simulink model "lab2"  (R2018b)
settings: Solver=VariableStepAuto  StartTime=0.0  StopTime=10.0  RelTol=1e-3
settings Model: Creator=grecu  LastModifiedBy=grecu

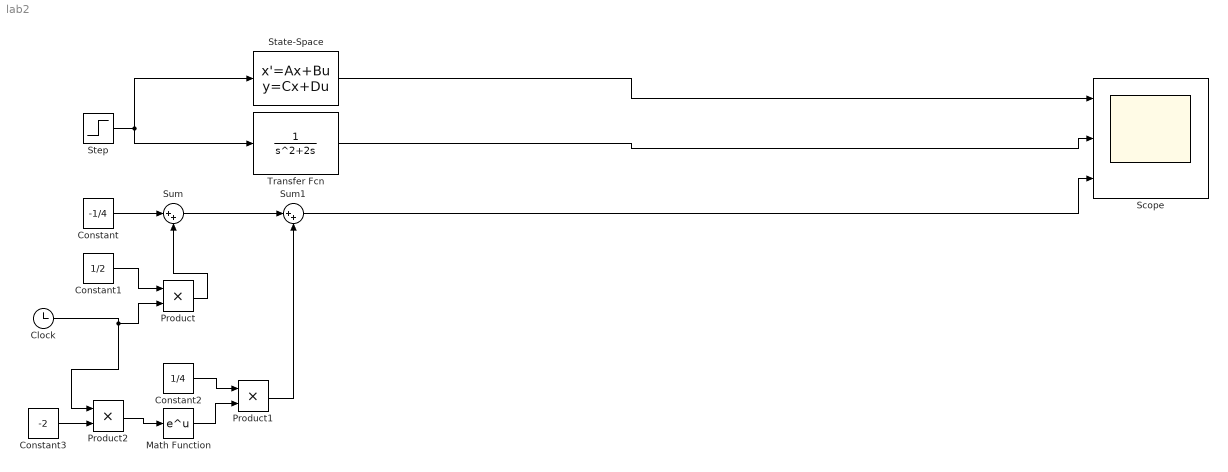
== system lab2 ==
  Clock : Clock
  Constant : Constant  Value=-1/4
  Constant1 : Constant  Value=1/2
  Constant2 : Constant  Value=1/4
  Constant3 : Constant  Value=-2
  Math Function : Math  SaturateOnIntegerOverflow=on
  Product : Product
  Product1 : Product
  Product2 : Product
  Scope : Scope  NumInputPorts=3
  State-Space : StateSpace  A=[-4,-4,0;1,0,0;0,1,0]  B=[1;0;0]  C=[0,1,2]  D=0  InitialCondition=0
  Step : Step  Time=0  SampleTime=0
  Sum : Sum  Inputs=|++
  Sum1 : Sum  Inputs=|++
  Transfer Fcn : TransferFcn  Denominator=[1 2 0]
  wires:
  Step/1 -> Transfer Fcn/1, State-Space/1
  Constant/1 -> Sum/1
  Constant1/1 -> Product/1
  Clock/1 -> Product2/1, Product/2
  Product/1 -> Sum/2
  Sum/1 -> Sum1/1
  Constant2/1 -> Product1/1
  Constant3/1 -> Product2/2
  Product2/1 -> Math Function/1
  Math Function/1 -> Product1/2
  Product1/1 -> Sum1/2
  Sum1/1 -> Scope/3
  State-Space/1 -> Scope/1
  Transfer Fcn/1 -> Scope/2
